simulink model "A03_L07_2_2014"  (R2021b)
settings: Solver=ode45  StartTime=0.0  StopTime=1440.0  RelTol=1e-3  EnableMultiTasking=on
values from neighbouring files (symbols this model uses):
  K = 0.08    [A04_L7_script.m]
  P = 1000    [A04_L7_script.m]
  T1 = 180    [A04_L7_script.m]
  T2 = 720    [A04_L7_script.m]
settings Model: Creator=User  LastModifiedBy=Adi
settings SolverCC: AlgebraicLoopSolver=TrustRegion
settings DataIOCC: LimitDataPoints=on  SaveFormat=Array  ReturnWorkspaceOutputs=off
settings OptimizationCC: LifeSpan=inf
settings DebuggingCC: SolverPrmCheckMsg=warning  SFUnexpectedBacktrackingDiag=warning  SFNoUnconditionalDefaultTransitionDiag=warning  SFMachineParentedDataDiag=warning  ArithmeticOperatorsInVariantConditions=warning
settings HardwareCC: ProdBitPerPointer=32  ProdBitPerSizeT=32  ProdBitPerPtrDiffT=32  ProdLargestAtomicFloat=None  ProdIntDivRoundTo=Undefined  ProdEndianess=Unspecified  ProdWordSize=32  ProdHWDeviceType=32-bit Generic
settings ModelReferenceCC: PropagateSignalLabelsOutOfModel=off
settings SFSimCC: SimUseLocalCustomCode=off  CustomCodeUndefinedFunction=UseInterfaceOnly
settings RTWCC: RTWUseLocalCustomCode=off
settings CodeAppCC: StateflowObjectComments=on
settings GRTTargetCC: TargetLangStandard=C89/C90 (ANSI)
settings ConfigComp: CovMetricSettings=dw  CovSaveCumulativeToWorkspaceVar=on  CovSaveSingleToWorkspaceVar=on  CovExternalEMLEnable=off  CovSFcnEnable=off

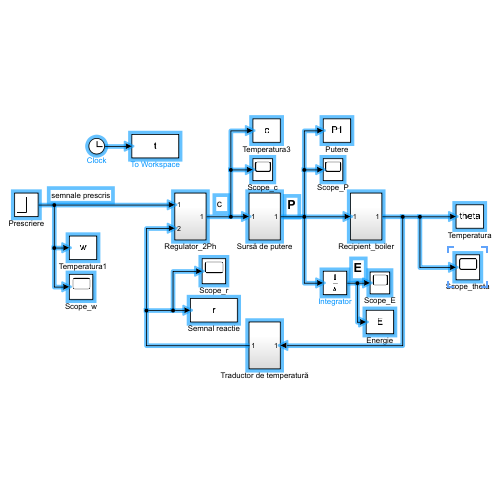
[thumbnail: Simulink's stored preview of the top-level diagram]
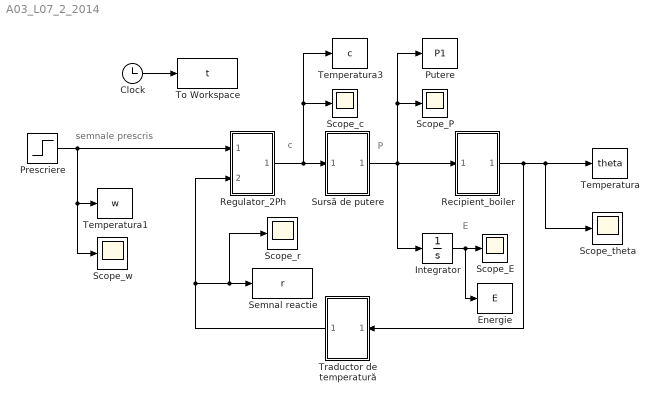
== system A03_L07_2_2014 ==
  note: semnale prescris
  note: c
  note: P
  note: E
  Clock : Clock
  Energie : ToWorkspace  VariableName=E  SampleTime=-1
  Integrator : Integrator
  Prescriere : Step  After=0.56  SampleTime=0
  Putere : ToWorkspace  VariableName=P1  SampleTime=-1
  Recipient_boiler : Subsystem
  Regulator_2Ph : Subsystem
  Scope_E : Scope
  Scope_P : Scope
  Scope_c : Scope
  Scope_r : Scope
  Scope_theta : Scope
  Scope_w : Scope
  Semnal reactie : ToWorkspace  VariableName=r  SampleTime=-1
  Sursă de putere : Subsystem
  Temperatura : ToWorkspace  VariableName=theta  SampleTime=-1
  Temperatura1 : ToWorkspace  VariableName=w  SampleTime=-1
  Temperatura3 : ToWorkspace  VariableName=c  SampleTime=-1
  To Workspace : ToWorkspace  VariableName=t  SampleTime=-1
  Traductor de temperatură : Subsystem
  wires:
  Prescriere/1 -> Scope_w/1, Temperatura1/1, Regulator_2Ph/1(In1)
  Clock/1 -> To Workspace/1
  Recipient_boiler/1(Out1) -> Traductor de temperatură/1(In1), Scope_theta/1, Temperatura/1
  Regulator_2Ph/1(Out1) -> Sursă de putere/1(In1), Temperatura3/1, Scope_c/1
  Traductor de temperatură/1(Out1) -> Regulator_2Ph/2(In2), Scope_r/1, Semnal reactie/1
  Integrator/1 -> Energie/1, Scope_E/1
  Sursă de putere/1(Out1) -> Integrator/1, Scope_P/1, Putere/1, Recipient_boiler/1(In1)

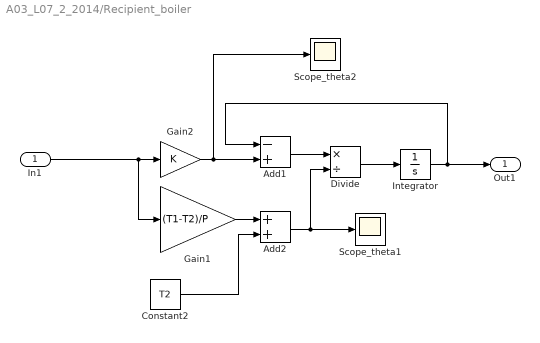
== system A03_L07_2_2014/Recipient_boiler ==
  In1 : Inport
  Add1 : Sum  Inputs=-+
  Add2 : Sum
  Constant2 : Constant  Value=T2
  Divide : Product  Inputs=*/
  Gain1 : Gain  Gain=(T1-T2)/P
  Gain2 : Gain  Gain=K
  Integrator : Integrator  InitialCondition=20
  Scope_theta1 : Scope
  Scope_theta2 : Scope
  Out1 : Outport
  wires:
  Divide/1 -> Integrator/1
  Add2/1 -> Scope_theta1/1, Divide/2
  In1/1 -> Gain1/1, Gain2/1
  Integrator/1 -> Out1/1, Add1/1
  Gain1/1 -> Add2/1
  Constant2/1 -> Add2/2
  Gain2/1 -> Scope_theta2/1, Add1/2
  Add1/1 -> Divide/1

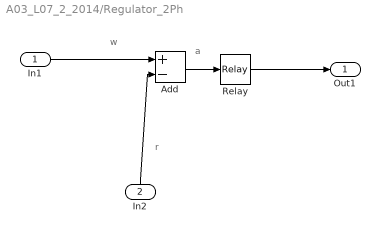
== system A03_L07_2_2014/Regulator_2Ph ==
  note: a
  note: r
  note: w
  In1 : Inport
  In2 : Inport  Port=2
  Add : Sum  Inputs=+-
  Relay : Relay  OnSwitchValue=0.03  OffSwitchValue=-0.03
  Out1 : Outport
  wires:
  Relay/1 -> Out1/1
  Add/1 -> Relay/1
  In1/1 -> Add/1
  In2/1 -> Add/2

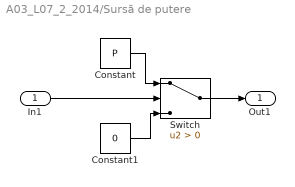
== system A03_L07_2_2014/Sursă de putere ==
  In1 : Inport
  Constant : Constant  Value=P
  Constant1 : Constant  Value=0
  Switch : Switch  Criteria=u2 > Threshold
  Out1 : Outport
  wires:
  Switch/1 -> Out1/1
  Constant/1 -> Switch/1
  In1/1 -> Switch/2
  Constant1/1 -> Switch/3

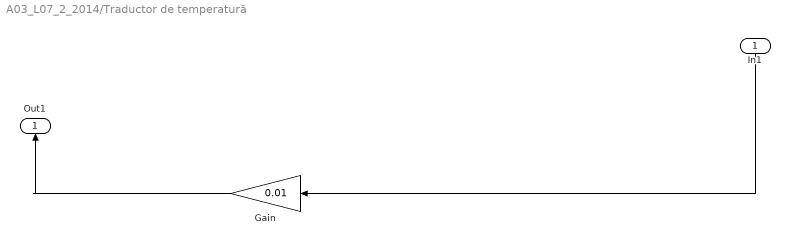
== system A03_L07_2_2014/Traductor de temperatură ==
  In1 : Inport
  Gain : Gain  Gain=0.01
  Out1 : Outport
  wires:
  Gain/1 -> Out1/1
  In1/1 -> Gain/1
